simulink model "h2p1_sim"  (R2021b)
settings: Solver=VariableStepAuto  StartTime=0.0  StopTime=Tf  RelTol=1e-3
undefined symbols (not defined in the file): J, mu, q_inertial2body_0, r_inertial_0, T, v_inertial_0, w_b_0
settings Model: Creator=corey  LastModifiedBy=corey

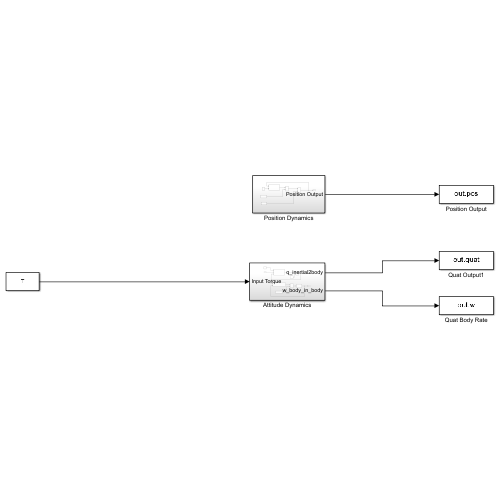
[thumbnail: Simulink's stored preview of the top-level diagram]
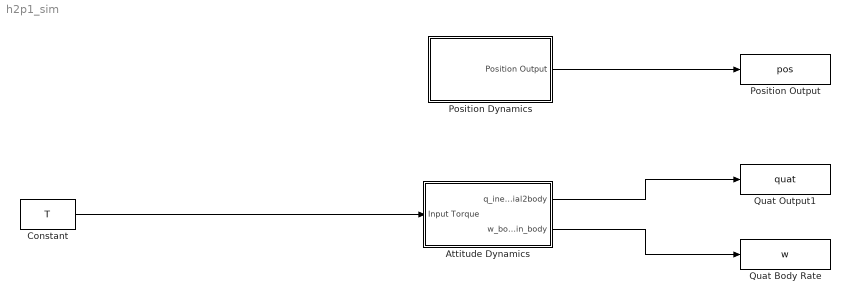
== system h2p1_sim ==
  Attitude Dynamics : Subsystem
  Constant : Constant  Value=T
  Position Dynamics : Subsystem
  Position Output : ToWorkspace  VariableName=pos  SampleTime=-1
  Quat Body Rate : ToWorkspace  VariableName=w  SampleTime=-1
  Quat Output1 : ToWorkspace  VariableName=quat  SampleTime=-1
  wires:
  Position Dynamics/1(Position Output) -> Position Output/1
  Constant/1 -> Attitude Dynamics/1(Input Torque)
  Attitude Dynamics/1(q_inertial2body) -> Quat Output1/1
  Attitude Dynamics/2(w_body_in_body) -> Quat Body Rate/1

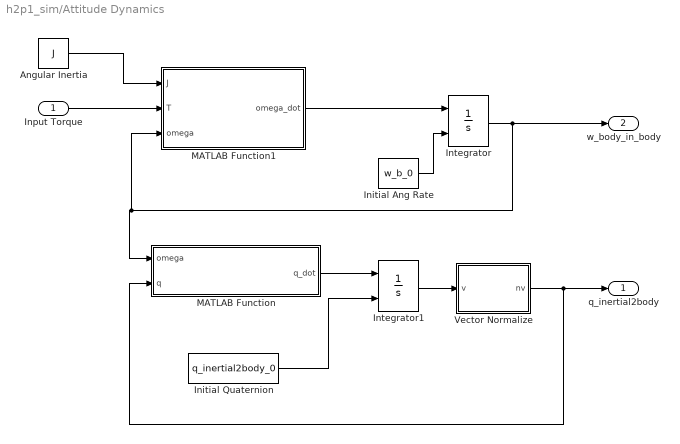
== system h2p1_sim/Attitude Dynamics ==
  Input Torque : Inport
  Angular Inertia : Constant  Value=J
  Initial Ang Rate : Constant  Value=w_b_0
  Initial Quaternion : Constant  Value=q_inertial2body_0
  Integrator : Integrator  InitialConditionSource=external
  Integrator1 : Integrator  InitialConditionSource=external
  MATLAB Function : MATLAB Function  TreatAsAtomicUnit=on
  MATLAB Function1 : MATLAB Function  TreatAsAtomicUnit=on
  Vector Normalize : MATLAB Function  TreatAsAtomicUnit=on
  q_inertial2body : Outport
  w_body_in_body : Outport  Port=2
  wires:
  Integrator/1 -> MATLAB Function1/3(omega), MATLAB Function/1(omega), w_body_in_body/1
  MATLAB Function1/1(omega_dot) -> Integrator/1
  Initial Ang Rate/1 -> Integrator/2
  MATLAB Function/1(q_dot) -> Integrator1/1
  Initial Quaternion/1 -> Integrator1/2
  Integrator1/1 -> Vector Normalize/1(v)
  Vector Normalize/1(nv) -> MATLAB Function/2(q), q_inertial2body/1
  Input Torque/1 -> MATLAB Function1/2(T)
  Angular Inertia/1 -> MATLAB Function1/1(J)

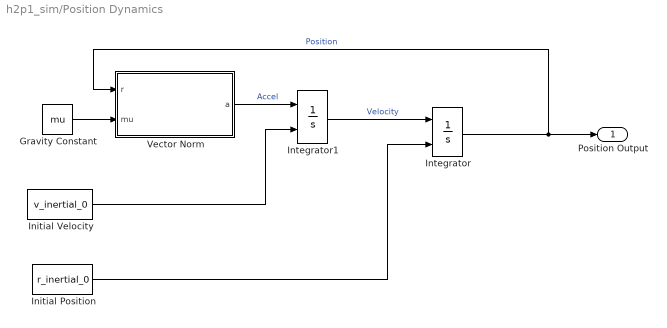
== system h2p1_sim/Position Dynamics ==
  Gravity Constant : Constant  Value=mu
  Initial Position : Constant  Value=r_inertial_0
  Initial Velocity : Constant  Value=v_inertial_0
  Integrator : Integrator  InitialConditionSource=external  InitialCondition=[6871, 0, 0]'
  Integrator1 : Integrator  InitialConditionSource=external  InitialCondition=[0, 7.6166, 0]'
  Vector Norm : MATLAB Function  TreatAsAtomicUnit=on
  Position Output : Outport
  wires:
  Integrator/1 -> Vector Norm/1(r), Position Output/1  "Position"
  Integrator1/1 -> Integrator/1  "Velocity"
  Vector Norm/1(a) -> Integrator1/1  "Accel"
  Gravity Constant/1 -> Vector Norm/2(mu)
  Initial Velocity/1 -> Integrator1/2
  Initial Position/1 -> Integrator/2

== matlab function h2p1_sim/Position Dynamics/Vector Norm ==
  data: r input; a output; mu input
function a = TwoBodyGrav(r,mu)

nr = norm(r);
a = -mu*r/(nr^3);

== matlab function h2p1_sim/Attitude Dynamics/MATLAB Function1 ==
  data: J input; omega_dot output; T input; omega input
function omega_dot = OmegaEvolution(J, T, omega)
omega_dot = J\(T - cross(omega, J*omega));

== matlab function h2p1_sim/Attitude Dynamics/Vector Normalize ==
  data: v input; nv output
function nv = NormVec(v)

nv = v/norm(v);

== matlab function h2p1_sim/Attitude Dynamics/MATLAB Function ==
  data: omega input; q_dot output; q input
function q_dot = QuaternionEvolution(omega, q)
intermed = [omega; 0];
q_dot = 0.5*QuatProduct(intermed,q);
